simulink model "VisionProcessingDesign_UCS"  (R2025b)
settings: Solver=FixedStepDiscrete  StartTime=0.0  StopTime=tspan  FixedStep=dt_sim  RelTol=1e-3
undefined symbols (not defined in the file): camHardwareDistK, dt_sample, gate1_Pose, M_WorldToUCS, pathPoses, redSlalomPoses, rel_CamPose_B, rel_CamPose_B_UCS, rel_CamPose_L, rel_CamPose_L_UCS, rel_CamPose_R, rel_CamPose_R_UCS, searchRescueEmojiPose, Sim3dSensor, surveyRepairEmojiPose, whiteSlalomPoses
libraries: sim3dlib x30, visionsinks x12, sim3dcameralib x3
settings Model: Creator=Liam  LastModifiedBy=Liam
settings OptimizationCC: DefaultParameterBehavior=Inlined  EnhancedBackFolding=on  PassReuseOutputArgsThreshold=0.0  ZeroExternalMemoryAtStartup=off  ZeroInternalMemoryAtStartup=off  InitFltsAndDblsToZero=on  OptimizeBlockOrder=speed  DifferentSizesBufferReuse=on  OptimizationCustomize=off
settings DebuggingCC: ParameterTunabilityLossMsg=error
settings HardwareCC: ProdLongLongMode=on  TargetLongLongMode=on
settings SFSimCC: SimTargetLang=C++  SimDLTargetLibrary=mkl-dnn
settings RTWCC: GenCodeOnly=on  GenerateReport=on  Toolchain=NVIDIA CUDA (w/Microsoft Visual C++ 2022) | nmake (64-bit Windows)  LaunchReport=on  TargetLang=C++  GenerateGPUCode=CUDA
settings CodeAppCC: ForceParamTrailComments=on  OperatorAnnotations=on
settings GRTTargetCC: TargetLangStandard=C++11 (ISO)  MatFileLogging=off  CodeInterfacePackaging=C++ class  SubcomponentCodeInterfacePackaging=C++ class

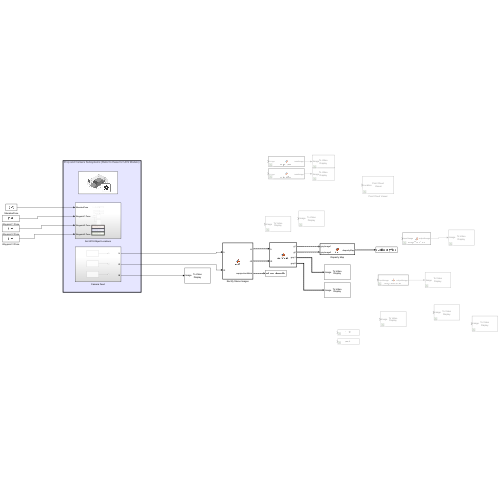
[thumbnail: Simulink's stored preview of the top-level diagram]
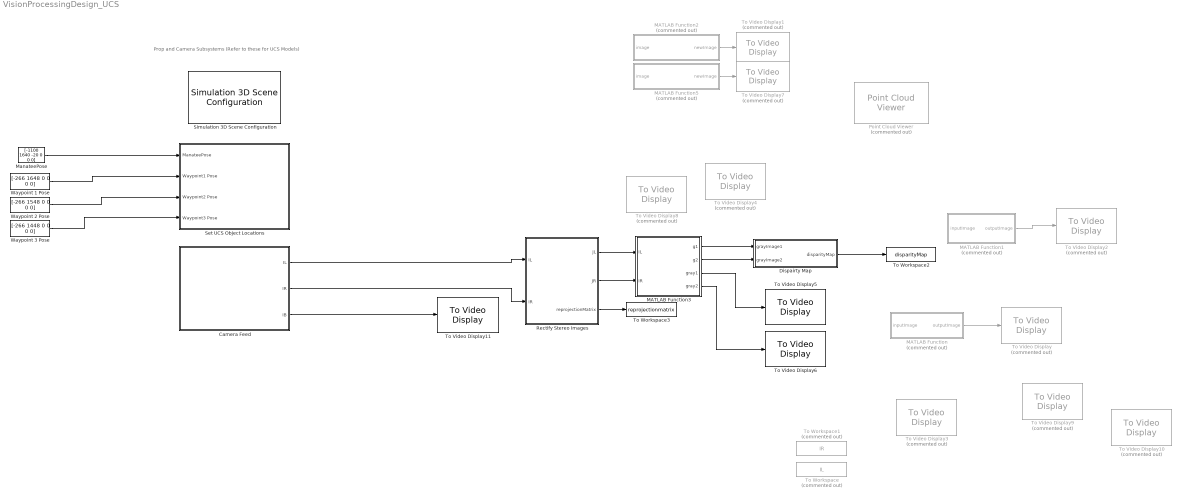
== system VisionProcessingDesign_UCS ==
  note: Prop and Camera Subsystems (Refer to these for UCS Models)
  Camera Feed : Subsystem  Priority=1
  Dispairty Map : MATLAB Function  TreatAsAtomicUnit=on
  MATLAB Function : MATLAB Function  Commented=on  TreatAsAtomicUnit=on
  MATLAB Function1 : MATLAB Function  Commented=on  TreatAsAtomicUnit=on
  MATLAB Function2 : MATLAB Function  Commented=on  TreatAsAtomicUnit=on
  MATLAB Function3 : MATLAB Function  TreatAsAtomicUnit=on
  MATLAB Function5 : MATLAB Function  Commented=on  TreatAsAtomicUnit=on
  ManateePose : Constant  Value=[-1100 1640 -20 0 0 0]
  Point Cloud Viewer : PointCloudViewer  Commented=on
  Rectify Stereo Images : MATLAB Function  TreatAsAtomicUnit=on
  Set UCS Object Locations : Subsystem  Priority=1
  Simulation 3D Scene Configuration : sim3dlib/Simulation 3D Scene Configuration  Priority=0  ProjectFormat=Unreal Executable  SceneDesc=Straight road  ProjectName=C:\Users\Liam\OneDrive\Documents\GitHub\SimulinkPlant\DROP UCS PACKAGED BUILD HERE\EllingtonPoolSim.exe  ScenePath=/Game/Olympic_Pool_Course  UEProjPath=C:\Users\Liam\OneDrive\Documents\GitHub\Vision_Sim\Unreal\UnrealProjects\SimulinkCoSimulation\EllingtonPoolSim\EllingtonPoolSim.uproject  EnableOpenDRIVE=off  vehTagList={'Custom';'Scene Origin'}  vehTag=Scene Origin  AttachedCameraRelativeTranslation=[0 0 0]  FreeCameraDefaultInitialTranslation=[-6, 0, 2]  AttachedCameraRelativeRotation=[0 0 0]  FreeCameraDefaultInitialRotation=[0, -15, 0]  ViewpointName=Custom  FreeCameraInitialTranslation=[0, 0, 0]  ViewpointTranslation=[0 0 0]  FreeCameraInitialRotation=[0, 0, 0]  ViewpointRotation=[0 0 0]  OpVisEn=off  Ts=dt_sample  EnableWindow=on  EnableRemoteAccess=off  EnableWeather=off  SunAzimuth=90  SunAltitude=40.0  EnableGeospatialSun=off  Latitude=0  Longitude=0  Date=2023-01-01  Time=10:30:00  GeoTimeZone=-5.0  SunDaylightSaving=off  wind=1  clouds=10  EnableVolumetricClouds=off  CloudCoverage=0  CloudAltitude=6  fog=0  rain=0  RaindropsEffect=off  SnowDensity=0  EnableGeospatial=off  TilesetSource=Earth terrain  UseTrueOrigin=off  OriginHeight=200  OriginLatitude=40.744652  OriginLongitude=-73.988864  MapStyle=Aerial  AdditionalAssetIDs=[]  UseAdvancedSunSky=off  SolarTime=11  TimeZone=-5  Day=21  Month=9  Year=2022  UseDaylightSavingTime=on  DSTStartDay=10  DSTStartMonth=3  DSTEndDay=3  DSTEndMonth=11  DSTSwitchHour=2  sensorTag=MainCamera1  sensorId=1  sensorName=MainCamera1  mountLoc=Origin  offsetFlag=off  tmountOffset=[0, 0, 0]  rmountOffset=[0, 0, 0]  HorizontalResolution=1280  VerticalResolution=720  HorizontalFOV=60  mountPoint=[0 0 0]  mountOrientation=[0 0 0]  aMode=3  ID=1  GeoTrigger=Inactive  ViewNameList={'Custom'}  ViewTranslationList={'[0 0 0]'}  ViewRotationList={'[0 0 0]'}
      settings: LibrarySourceBlock=drivingsim3d/Simulation 3D Scene Configuration
  To Video Display{,1..3,7,9..10} (7 alike) : visionsinks/To Video Display  Commented=on  windowSizeMode=Normal  openAtMdlStart=on  fullScreen=off  videoWindowX=536805376  videoWindowY=536805376  saveWindowSize=off  videoWindowWidth=1920  videoWindowHeight=1080  inputColorFormat=RGB  inputType=Obsolete  imagePorts=One multidimensional signal  OutputDevice=On-screen video monitor  dataOrg=Column-major  isWindowOpen=off
  To Video Display11 : visionsinks/To Video Display  windowSizeMode=Normal  openAtMdlStart=on  fullScreen=off  videoWindowX=536805376  videoWindowY=536805376  saveWindowSize=off  videoWindowWidth=1920  videoWindowHeight=1080  inputColorFormat=RGB  inputType=Obsolete  imagePorts=One multidimensional signal  OutputDevice=On-screen video monitor  dataOrg=Column-major  isWindowOpen=off
  To Video Display4 : visionsinks/To Video Display  Commented=on  windowSizeMode=Normal  openAtMdlStart=on  fullScreen=off  videoWindowX=536805376  videoWindowY=536805376  saveWindowSize=off  videoWindowWidth=1491  videoWindowHeight=834  inputColorFormat=RGB  inputType=Obsolete  imagePorts=One multidimensional signal  OutputDevice=On-screen video monitor  dataOrg=Column-major  isWindowOpen=off
  To Video Display5 : visionsinks/To Video Display  windowSizeMode=Normal  openAtMdlStart=on  fullScreen=off  videoWindowX=536805376  videoWindowY=536805376  saveWindowSize=off  videoWindowWidth=1491  videoWindowHeight=834  inputColorFormat=RGB  inputType=Obsolete  imagePorts=One multidimensional signal  OutputDevice=On-screen video monitor  dataOrg=Column-major  isWindowOpen=off
  To Video Display6 : visionsinks/To Video Display  windowSizeMode=Normal  openAtMdlStart=on  fullScreen=off  videoWindowX=536805376  videoWindowY=536805376  saveWindowSize=off  videoWindowWidth=1491  videoWindowHeight=834  inputColorFormat=RGB  inputType=Obsolete  imagePorts=One multidimensional signal  OutputDevice=On-screen video monitor  dataOrg=Column-major  isWindowOpen=off
  To Video Display8 : visionsinks/To Video Display  Commented=on  windowSizeMode=Normal  openAtMdlStart=on  fullScreen=off  videoWindowX=536805376  videoWindowY=536805376  saveWindowSize=off  videoWindowWidth=1491  videoWindowHeight=834  inputColorFormat=RGB  inputType=Obsolete  imagePorts=One multidimensional signal  OutputDevice=On-screen video monitor  dataOrg=Column-major  isWindowOpen=off
  To Workspace : ToWorkspace  Commented=on  VariableName=IL  SaveFormat=Structure  SampleTime=-1
  To Workspace1 : ToWorkspace  Commented=on  VariableName=IR  SaveFormat=Structure  SampleTime=-1
  To Workspace2 : ToWorkspace  VariableName=disparityMap  SaveFormat=Structure  SampleTime=-1
  To Workspace3 : ToWorkspace  VariableName=reprojectionmatrix  SaveFormat=Structure  SampleTime=-1
  Waypoint 1 Pose : Constant  Value=[-266 1648 0 0 0 0]
  Waypoint 2 Pose : Constant  Value=[-266 1548 0 0 0 0]
  Waypoint 3 Pose : Constant  Value=[-266 1448 0 0 0 0]
  wires:
  ManateePose/1 -> Set UCS Object Locations/1(ManateePose)
  MATLAB Function/1(outputImage) -> To Video Display/1
  MATLAB Function1/1(outputImage) -> To Video Display2/1
  MATLAB Function2/1(newImage) -> To Video Display1/1
  MATLAB Function5/1(newImage) -> To Video Display7/1
  Camera Feed/1(IL) -> Rectify Stereo Images/1(IL)
  Camera Feed/2(IR) -> Rectify Stereo Images/2(IR)
  Camera Feed/3(IB) -> To Video Display11/1
  Waypoint 1 Pose/1 -> Set UCS Object Locations/2(Waypoint1 Pose)
  Waypoint 2 Pose/1 -> Set UCS Object Locations/3(Waypoint2 Pose)
  Waypoint 3 Pose/1 -> Set UCS Object Locations/4(Waypoint3 Pose)
  MATLAB Function3/2(g2) -> Dispairty Map/2(grayImage2)
  Rectify Stereo Images/1(JL) -> MATLAB Function3/1(IL)
  MATLAB Function3/1(g1) -> Dispairty Map/1(grayImage1)
  Rectify Stereo Images/2(JR) -> MATLAB Function3/2(IR)
  Dispairty Map/1(disparityMap) -> To Workspace2/1
  MATLAB Function3/3(gray1) -> To Video Display5/1
  MATLAB Function3/4(gray2) -> To Video Display6/1
  Rectify Stereo Images/3(reprojectionMatrix) -> To Workspace3/1

== system VisionProcessingDesign_UCS/Camera Feed ==
  Simulation 3D Manatee Bottom Camera : sim3dcameralib/Simulation 3D Camera  Priority=1  sensorTag=Sim3dSensor�  sensorId=1  sensorName=Sim3dSensor�  vehTagList={'Scene Origin'}  vehTag=Scene Origin  CoordinateSystem=Default  mountLoc=Origin  offsetFlag=on  tmountOffset=rel_CamPose_B_UCS(1:3) / 100  extTmount=off  rmountOffset=rel_CamPose_B(4:6)  extRmount=off  FocalLength=[2.97 / 0.0028, 2.97 / 0.0028]  OpticalCenter=[960, 540]  ImageSize=[1080, 1920]  RadialDistortion=[camHardwareDistK(1) camHardwareDistK(2) camHardwareDistK(5)]  TangentialDistortion=[camHardwareDistK(3) camHardwareDistK(4)]  SensorSkew=0  VisualizeFieldOfView=on  FieldOfViewRange=61  DepthOutportEnabled=off  SemanticOutportEnabled=off  TransformOutportEnabled=off  SampleTime=dt_sample  mountPoint=[0.23 0 -0.08]  mountOrientation=[0 -1.5707963267949 0]  aMode=5  ID=1
      settings: LibrarySourceBlock=sl3dlib/Simulation 3D/Sensors/Simulation 3D Camera
  Simulation 3D Manatee Left Camera : sim3dcameralib/Simulation 3D Camera  Priority=1  sensorTag=Sim3dSensor�  sensorId=2  sensorName=Sim3dSensor�  vehTagList={'Scene Origin'}  vehTag=Scene Origin  CoordinateSystem=Default  mountLoc=Origin  offsetFlag=on  tmountOffset=rel_CamPose_L_UCS(1:3) / 100  extTmount=off  rmountOffset=rel_CamPose_L(4:6)  extRmount=off  FocalLength=[2.97 / 0.0028, 2.97 / 0.0028]  OpticalCenter=[960, 540]  ImageSize=[1080, 1920]  RadialDistortion=[camHardwareDistK(1) camHardwareDistK(2) camHardwareDistK(5)]  TangentialDistortion=[camHardwareDistK(3) camHardwareDistK(4)]  SensorSkew=0  VisualizeFieldOfView=on  FieldOfViewRange=61  DepthOutportEnabled=off  SemanticOutportEnabled=off  TransformOutportEnabled=off  SampleTime=dt_sample  mountPoint=[0.38 -0.024 0.14]  mountOrientation=[0 0 0]  aMode=5  ID=2
      settings: LibrarySourceBlock=sl3dlib/Simulation 3D/Sensors/Simulation 3D Camera
  Simulation 3D Manatee Right Camera : sim3dcameralib/Simulation 3D Camera  Priority=1  sensorTag=Sim3dSensor�  sensorId=3  sensorName=Sim3dSensor�  vehTagList={'Scene Origin'}  vehTag=Scene Origin  CoordinateSystem=Default  mountLoc=Origin  offsetFlag=on  tmountOffset=rel_CamPose_R_UCS(1:3) / 100  extTmount=off  rmountOffset=rel_CamPose_R(4:6)  extRmount=off  FocalLength=[2.97 / 0.0028, 2.97 / 0.0028]  OpticalCenter=[960, 540]  ImageSize=[1080, 1920]  RadialDistortion=[camHardwareDistK(1) camHardwareDistK(2) camHardwareDistK(5)]  TangentialDistortion=[camHardwareDistK(3) camHardwareDistK(4)]  SensorSkew=0  VisualizeFieldOfView=on  FieldOfViewRange=61  DepthOutportEnabled=off  SemanticOutportEnabled=off  TransformOutportEnabled=off  SampleTime=dt_sample  mountPoint=[0.38 0.024 0.14]  mountOrientation=[0 0 0]  aMode=5  ID=3
      settings: LibrarySourceBlock=sl3dlib/Simulation 3D/Sensors/Simulation 3D Camera
  IL : Outport
  IR : Outport  Port=2
  IB : Outport  Port=3
  wires:
  Simulation 3D Manatee Left Camera/1 -> IL/1
  Simulation 3D Manatee Right Camera/1 -> IR/1
  Simulation 3D Manatee Bottom Camera/1 -> IB/1

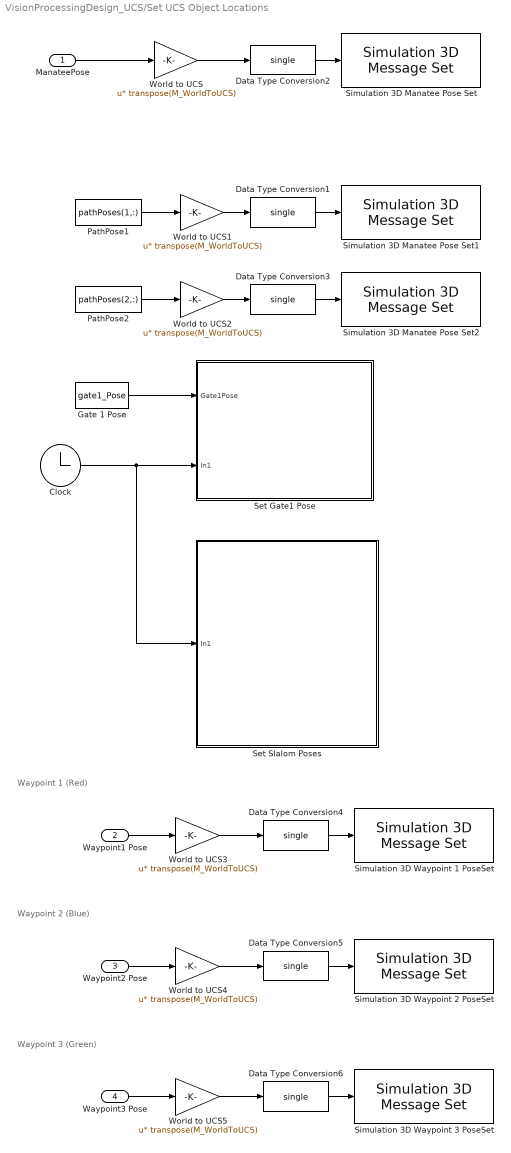
== system VisionProcessingDesign_UCS/Set UCS Object Locations ==
  note: Waypoint 1 (Red)
  note: Waypoint 2 (Blue)
  note: Waypoint 3 (Green)
  ManateePose : Inport
  Waypoint1 Pose : Inport  Port=2
  Waypoint2 Pose : Inport  Port=3
  Waypoint3 Pose : Inport  Port=4
  Clock : Clock
      settings: Decimation=dt_sample/dt_sim
  Data Type Conversion{1..6} (6 alike) : DataTypeConversion  OutDataTypeStr=single  SaturateOnIntegerOverflow=off  RndMeth=Floor
  Gate 1 Pose : Constant  Value=gate1_Pose
  PathPose1 : Constant  Value=pathPoses(1,:)
  PathPose2 : Constant  Value=pathPoses(2,:)
  Set Gate1 Pose : Subsystem
  Set Slalom Poses : Subsystem
  Simulation 3D Manatee Pose Set : sim3dlib/Simulation 3D Message Set  Priority=-1  SigName=ManateePoseSet  Ts=dt_sample  aMode=0
      settings: LibrarySourceBlock=aerolibsim3d/Simulation 3D Message Set
  Simulation 3D Manatee Pose Set1 : sim3dlib/Simulation 3D Message Set  Priority=-1  SigName=Path1PoseSet  Ts=dt_sample  aMode=0
      settings: LibrarySourceBlock=aerolibsim3d/Simulation 3D Message Set
  Simulation 3D Manatee Pose Set2 : sim3dlib/Simulation 3D Message Set  Priority=-1  SigName=Path2PoseSet  Ts=dt_sample  aMode=0
      settings: LibrarySourceBlock=aerolibsim3d/Simulation 3D Message Set
  Simulation 3D Waypoint 1 PoseSet : sim3dlib/Simulation 3D Message Set  Priority=-1  SigName=Waypoint1PoseSet  Ts=dt_sample  aMode=0
      settings: LibrarySourceBlock=aerolibsim3d/Simulation 3D Message Set
  Simulation 3D Waypoint 2 PoseSet : sim3dlib/Simulation 3D Message Set  Priority=-1  SigName=Waypoint2PoseSet  Ts=dt_sample  aMode=0
      settings: LibrarySourceBlock=aerolibsim3d/Simulation 3D Message Set
  Simulation 3D Waypoint 3 PoseSet : sim3dlib/Simulation 3D Message Set  Priority=-1  SigName=Waypoint3PoseSet  Ts=dt_sample  aMode=0
      settings: LibrarySourceBlock=aerolibsim3d/Simulation 3D Message Set
  World to UCS{,1..5} (6 alike) : Gain  Gain=transpose(M_WorldToUCS)  Multiplication=Matrix(u*K)
  wires:
  Gate 1 Pose/1 -> Set Gate1 Pose/1(Gate1Pose)
  Data Type Conversion2/1 -> Simulation 3D Manatee Pose Set/1
  World to UCS1/1 -> Data Type Conversion1/1
  Data Type Conversion1/1 -> Simulation 3D Manatee Pose Set1/1
  PathPose1/1 -> World to UCS1/1
  World to UCS2/1 -> Data Type Conversion3/1
  Data Type Conversion3/1 -> Simulation 3D Manatee Pose Set2/1
  PathPose2/1 -> World to UCS2/1
  Clock/1 -> Set Slalom Poses/1(In1), Set Gate1 Pose/2(In1)
  World to UCS/1 -> Data Type Conversion2/1
  ManateePose/1 -> World to UCS/1
  Waypoint1 Pose/1 -> World to UCS3/1
  Data Type Conversion4/1 -> Simulation 3D Waypoint 1 PoseSet/1
  World to UCS3/1 -> Data Type Conversion4/1
  Waypoint2 Pose/1 -> World to UCS4/1
  Data Type Conversion5/1 -> Simulation 3D Waypoint 2 PoseSet/1
  World to UCS4/1 -> Data Type Conversion5/1
  World to UCS5/1 -> Data Type Conversion6/1
  Waypoint3 Pose/1 -> World to UCS5/1
  Data Type Conversion6/1 -> Simulation 3D Waypoint 3 PoseSet/1

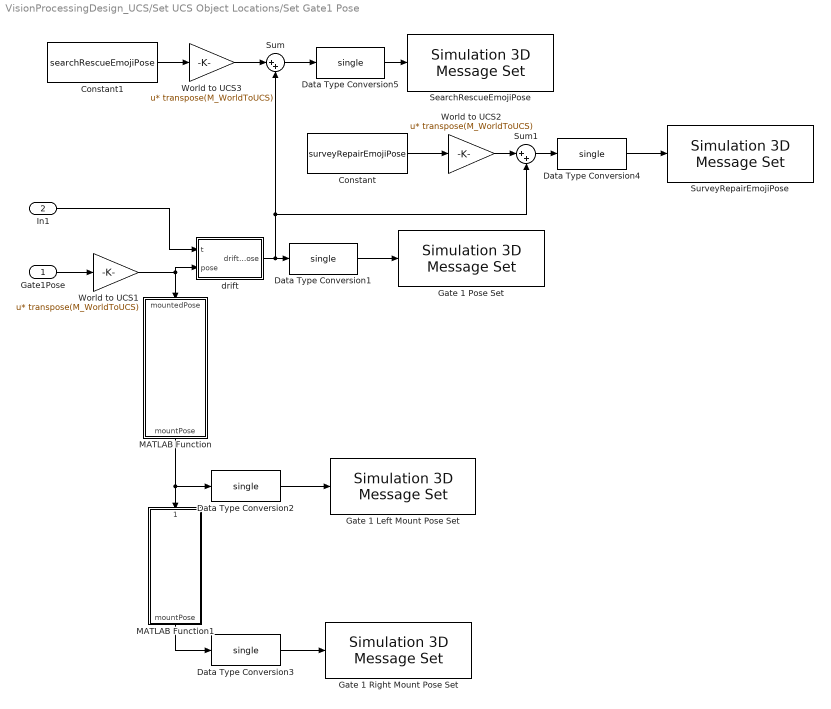
== system VisionProcessingDesign_UCS/Set UCS Object Locations/Set Gate1 Pose ==
  Gate1Pose : Inport
  In1 : Inport  Port=2
  Constant : Constant  Value=surveyRepairEmojiPose
  Constant1 : Constant  Value=searchRescueEmojiPose
  Data Type Conversion{1..5} (5 alike) : DataTypeConversion  OutDataTypeStr=single  SaturateOnIntegerOverflow=off  RndMeth=Floor
  Gate 1 Left Mount Pose Set : sim3dlib/Simulation 3D Message Set  Priority=-1  SigName=Gate1LeftMountPoseSet  Ts=dt_sample  aMode=0
      settings: LibrarySourceBlock=aerolibsim3d/Simulation 3D Message Set
  Gate 1 Pose Set : sim3dlib/Simulation 3D Message Set  Priority=-1  SigName=Gate1PoseSet  Ts=dt_sample  aMode=0
      settings: LibrarySourceBlock=aerolibsim3d/Simulation 3D Message Set
  Gate 1 Right Mount Pose Set : sim3dlib/Simulation 3D Message Set  Priority=-1  SigName=Gate1RightMountPoseSet  Ts=dt_sample  aMode=0
      settings: LibrarySourceBlock=aerolibsim3d/Simulation 3D Message Set
  MATLAB Function : MATLAB Function  TreatAsAtomicUnit=on
  MATLAB Function1 : MATLAB Function  TreatAsAtomicUnit=on
  SearchRescueEmojiPose : sim3dlib/Simulation 3D Message Set  Priority=-1  SigName=SearchRescueEmojiPoseSet  Ts=dt_sample  aMode=0
      settings: LibrarySourceBlock=aerolibsim3d/Simulation 3D Message Set
  Sum : Sum  Inputs=|++
  Sum1 : Sum  Inputs=|++
  SurveyRepairEmojiPose : sim3dlib/Simulation 3D Message Set  Priority=-1  SigName=SurveyRepairEmojiPoseSet  Ts=dt_sample  aMode=0
      settings: LibrarySourceBlock=aerolibsim3d/Simulation 3D Message Set
  World to UCS1 : Gain  Gain=transpose(M_WorldToUCS)  Multiplication=Matrix(u*K)
  World to UCS2 : Gain  Gain=transpose(M_WorldToUCS)  Multiplication=Matrix(u*K)
  World to UCS3 : Gain  Gain=transpose(M_WorldToUCS)  Multiplication=Matrix(u*K)
  drift : MATLAB Function  TreatAsAtomicUnit=on
  wires:
  Gate1Pose/1 -> World to UCS1/1
  MATLAB Function/1(mountPose) -> Data Type Conversion2/1, MATLAB Function1/1(leftMountPose)
  Data Type Conversion2/1 -> Gate 1 Left Mount Pose Set/1
  Data Type Conversion3/1 -> Gate 1 Right Mount Pose Set/1
  Data Type Conversion1/1 -> Gate 1 Pose Set/1
  World to UCS1/1 -> drift/2(pose), MATLAB Function/1(mountedPose)
  MATLAB Function1/1(mountPose) -> Data Type Conversion3/1
  Data Type Conversion4/1 -> SurveyRepairEmojiPose/1
  Constant/1 -> World to UCS2/1
  Data Type Conversion5/1 -> SearchRescueEmojiPose/1
  Constant1/1 -> World to UCS3/1
  Sum/1 -> Data Type Conversion5/1
  World to UCS3/1 -> Sum/1
  World to UCS2/1 -> Sum1/1
  Sum1/1 -> Data Type Conversion4/1
  In1/1 -> drift/1(t)
  drift/1(driftPose) -> Data Type Conversion1/1, Sum1/2, Sum/2

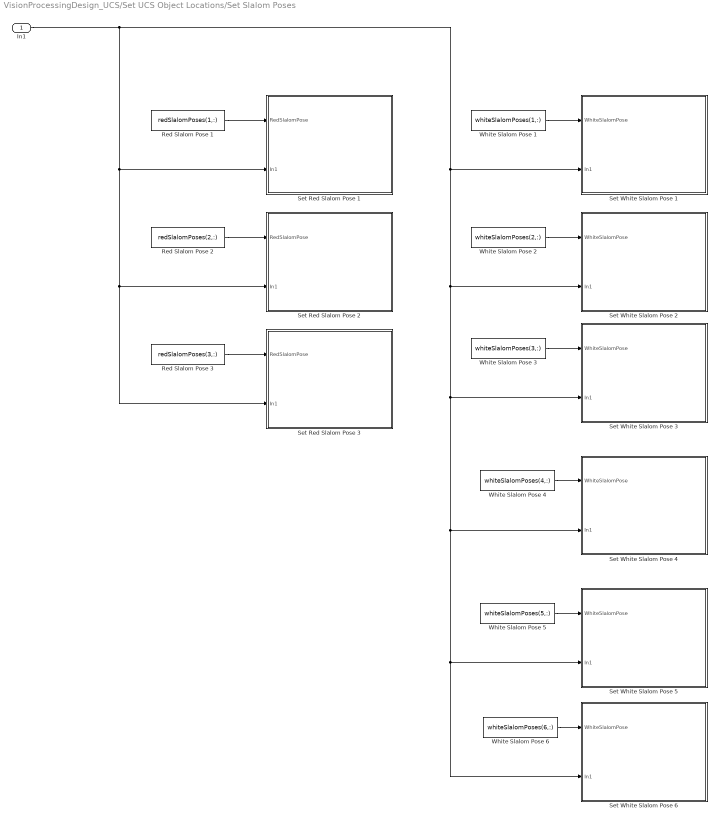
== system VisionProcessingDesign_UCS/Set UCS Object Locations/Set Slalom Poses ==
  In1 : Inport
  Red Slalom Pose 1 : Constant  Value=redSlalomPoses(1,:)
  Red Slalom Pose 2 : Constant  Value=redSlalomPoses(2,:)
  Red Slalom Pose 3 : Constant  Value=redSlalomPoses(3,:)
  Set Red Slalom Pose 1 : Subsystem
  Set Red Slalom Pose 2 : Subsystem
  Set Red Slalom Pose 3 : Subsystem
  Set White Slalom Pose 1 : Subsystem
  Set White Slalom Pose 2 : Subsystem
  Set White Slalom Pose 3 : Subsystem
  Set White Slalom Pose 4 : Subsystem
  Set White Slalom Pose 5 : Subsystem
  Set White Slalom Pose 6 : Subsystem
  White Slalom Pose 1 : Constant  Value=whiteSlalomPoses(1,:)
  White Slalom Pose 2 : Constant  Value=whiteSlalomPoses(2,:)
  White Slalom Pose 3 : Constant  Value=whiteSlalomPoses(3,:)
  White Slalom Pose 4 : Constant  Value=whiteSlalomPoses(4,:)
  White Slalom Pose 5 : Constant  Value=whiteSlalomPoses(5,:)
  White Slalom Pose 6 : Constant  Value=whiteSlalomPoses(6,:)
  wires:
  Red Slalom Pose 1/1 -> Set Red Slalom Pose 1/1(RedSlalomPose)
  Red Slalom Pose 2/1 -> Set Red Slalom Pose 2/1(RedSlalomPose)
  Red Slalom Pose 3/1 -> Set Red Slalom Pose 3/1(RedSlalomPose)
  White Slalom Pose 1/1 -> Set White Slalom Pose 1/1(WhiteSlalomPose)
  White Slalom Pose 2/1 -> Set White Slalom Pose 2/1(WhiteSlalomPose)
  White Slalom Pose 3/1 -> Set White Slalom Pose 3/1(WhiteSlalomPose)
  White Slalom Pose 4/1 -> Set White Slalom Pose 4/1(WhiteSlalomPose)
  White Slalom Pose 5/1 -> Set White Slalom Pose 5/1(WhiteSlalomPose)
  White Slalom Pose 6/1 -> Set White Slalom Pose 6/1(WhiteSlalomPose)
  In1/1 -> Set Red Slalom Pose 3/2(In1), Set Red Slalom Pose 2/2(In1), Set Red Slalom Pose 1/2(In1), Set White Slalom Pose 6/2(In1), Set White Slalom Pose 5/2(In1), Set White Slalom Pose 4/2(In1), Set White Slalom Pose 3/2(In1), Set White Slalom Pose 2/2(In1), Set White Slalom Pose 1/2(In1)

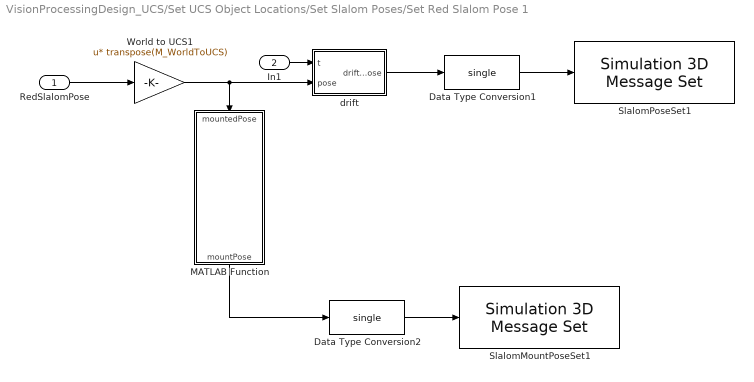
== system VisionProcessingDesign_UCS/Set UCS Object Locations/Set Slalom Poses/Set Red Slalom Pose 1 ==
  RedSlalomPose : Inport
  In1 : Inport  Port=2
  Data Type Conversion1 : DataTypeConversion  OutDataTypeStr=single  SaturateOnIntegerOverflow=off  RndMeth=Floor
  Data Type Conversion2 : DataTypeConversion  OutDataTypeStr=single  SaturateOnIntegerOverflow=off  RndMeth=Floor
  MATLAB Function : MATLAB Function  TreatAsAtomicUnit=on
  SlalomMountPoseSet1 : sim3dlib/Simulation 3D Message Set  Priority=-1  SigName=RedSlalom1MountPoseSet  Ts=dt_sample  aMode=0
      settings: LibrarySourceBlock=aerolibsim3d/Simulation 3D Message Set
  SlalomPoseSet1 : sim3dlib/Simulation 3D Message Set  Priority=-1  SigName=RedSlalom1PoseSet  Ts=dt_sample  aMode=0
      settings: LibrarySourceBlock=aerolibsim3d/Simulation 3D Message Set
  World to UCS1 : Gain  Gain=transpose(M_WorldToUCS)  Multiplication=Matrix(u*K)
  drift : MATLAB Function  TreatAsAtomicUnit=on
  wires:
  RedSlalomPose/1 -> World to UCS1/1
  MATLAB Function/1(mountPose) -> Data Type Conversion2/1
  Data Type Conversion2/1 -> SlalomMountPoseSet1/1
  Data Type Conversion1/1 -> SlalomPoseSet1/1
  World to UCS1/1 -> drift/2(pose), MATLAB Function/1(mountedPose)
  drift/1(driftPose) -> Data Type Conversion1/1
  In1/1 -> drift/1(t)

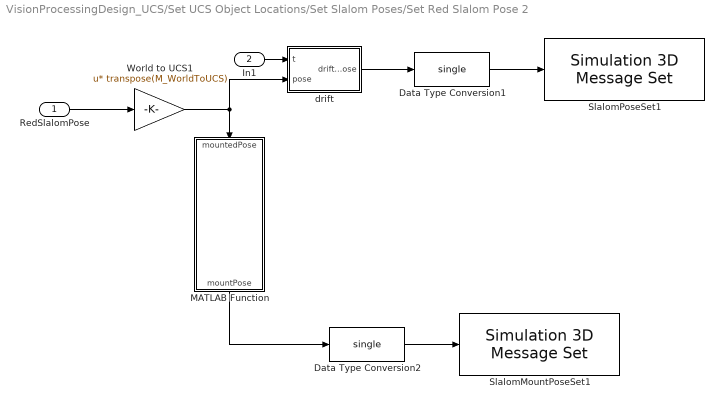
== system VisionProcessingDesign_UCS/Set UCS Object Locations/Set Slalom Poses/Set Red Slalom Pose 2 ==
  RedSlalomPose : Inport
  In1 : Inport  Port=2
  Data Type Conversion1 : DataTypeConversion  OutDataTypeStr=single  SaturateOnIntegerOverflow=off  RndMeth=Floor
  Data Type Conversion2 : DataTypeConversion  OutDataTypeStr=single  SaturateOnIntegerOverflow=off  RndMeth=Floor
  MATLAB Function : MATLAB Function  TreatAsAtomicUnit=on
  SlalomMountPoseSet1 : sim3dlib/Simulation 3D Message Set  Priority=-1  SigName=RedSlalom2MountPoseSet  Ts=dt_sample  aMode=0
      settings: LibrarySourceBlock=aerolibsim3d/Simulation 3D Message Set
  SlalomPoseSet1 : sim3dlib/Simulation 3D Message Set  Priority=-1  SigName=RedSlalom2PoseSet  Ts=dt_sample  aMode=0
      settings: LibrarySourceBlock=aerolibsim3d/Simulation 3D Message Set
  World to UCS1 : Gain  Gain=transpose(M_WorldToUCS)  Multiplication=Matrix(u*K)
  drift : MATLAB Function  TreatAsAtomicUnit=on
  wires:
  RedSlalomPose/1 -> World to UCS1/1
  MATLAB Function/1(mountPose) -> Data Type Conversion2/1
  Data Type Conversion2/1 -> SlalomMountPoseSet1/1
  Data Type Conversion1/1 -> SlalomPoseSet1/1
  World to UCS1/1 -> MATLAB Function/1(mountedPose), drift/2(pose)
  In1/1 -> drift/1(t)
  drift/1(driftPose) -> Data Type Conversion1/1

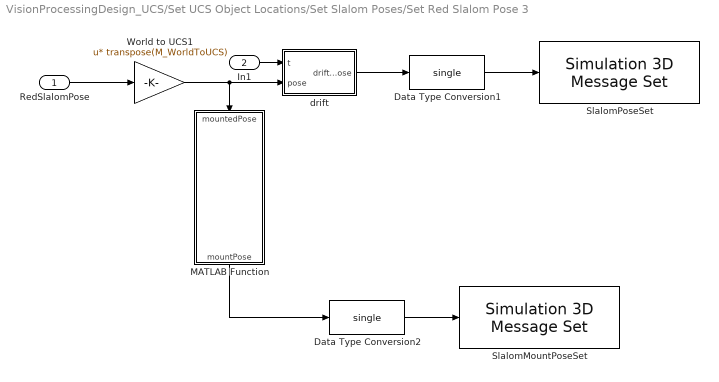
== system VisionProcessingDesign_UCS/Set UCS Object Locations/Set Slalom Poses/Set Red Slalom Pose 3 ==
  RedSlalomPose : Inport
  In1 : Inport  Port=2
  Data Type Conversion1 : DataTypeConversion  OutDataTypeStr=single  SaturateOnIntegerOverflow=off  RndMeth=Floor
  Data Type Conversion2 : DataTypeConversion  OutDataTypeStr=single  SaturateOnIntegerOverflow=off  RndMeth=Floor
  MATLAB Function : MATLAB Function  TreatAsAtomicUnit=on
  SlalomMountPoseSet : sim3dlib/Simulation 3D Message Set  Priority=-1  SigName=RedSlalom3MountPoseSet  Ts=dt_sample  aMode=0
      settings: LibrarySourceBlock=aerolibsim3d/Simulation 3D Message Set
  SlalomPoseSet : sim3dlib/Simulation 3D Message Set  Priority=-1  SigName=RedSlalom3PoseSet  Ts=dt_sample  aMode=0
      settings: LibrarySourceBlock=aerolibsim3d/Simulation 3D Message Set
  World to UCS1 : Gain  Gain=transpose(M_WorldToUCS)  Multiplication=Matrix(u*K)
  drift : MATLAB Function  TreatAsAtomicUnit=on
  wires:
  RedSlalomPose/1 -> World to UCS1/1
  MATLAB Function/1(mountPose) -> Data Type Conversion2/1
  Data Type Conversion2/1 -> SlalomMountPoseSet/1
  Data Type Conversion1/1 -> SlalomPoseSet/1
  World to UCS1/1 -> drift/2(pose), MATLAB Function/1(mountedPose)
  In1/1 -> drift/1(t)
  drift/1(driftPose) -> Data Type Conversion1/1

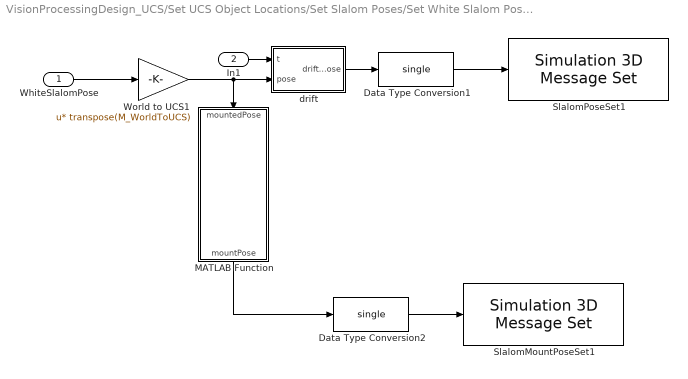
== system VisionProcessingDesign_UCS/Set UCS Object Locations/Set Slalom Poses/Set White Slalom Pose 1 ==
  WhiteSlalomPose : Inport
  In1 : Inport  Port=2
  Data Type Conversion1 : DataTypeConversion  OutDataTypeStr=single  SaturateOnIntegerOverflow=off  RndMeth=Floor
  Data Type Conversion2 : DataTypeConversion  OutDataTypeStr=single  SaturateOnIntegerOverflow=off  RndMeth=Floor
  MATLAB Function : MATLAB Function  TreatAsAtomicUnit=on
  SlalomMountPoseSet1 : sim3dlib/Simulation 3D Message Set  Priority=-1  SigName=WhiteSlalom1MountPoseSet  Ts=dt_sample  aMode=0
      settings: LibrarySourceBlock=aerolibsim3d/Simulation 3D Message Set
  SlalomPoseSet1 : sim3dlib/Simulation 3D Message Set  Priority=-1  SigName=WhiteSlalom1PoseSet  Ts=dt_sample  aMode=0
      settings: LibrarySourceBlock=aerolibsim3d/Simulation 3D Message Set
  World to UCS1 : Gain  Gain=transpose(M_WorldToUCS)  Multiplication=Matrix(u*K)
  drift : MATLAB Function  TreatAsAtomicUnit=on
  wires:
  WhiteSlalomPose/1 -> World to UCS1/1
  MATLAB Function/1(mountPose) -> Data Type Conversion2/1
  Data Type Conversion2/1 -> SlalomMountPoseSet1/1
  Data Type Conversion1/1 -> SlalomPoseSet1/1
  World to UCS1/1 -> drift/2(pose), MATLAB Function/1(mountedPose)
  In1/1 -> drift/1(t)
  drift/1(driftPose) -> Data Type Conversion1/1

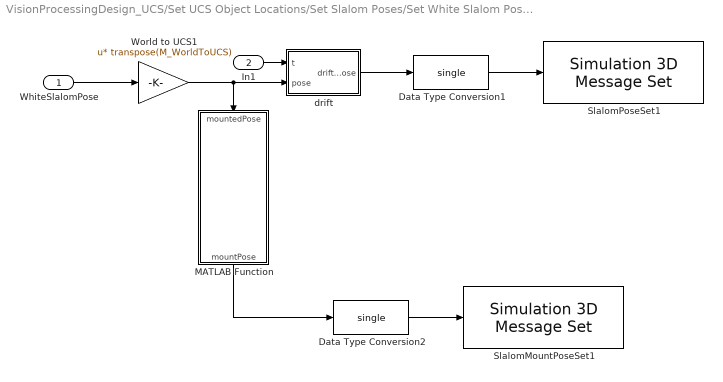
== system VisionProcessingDesign_UCS/Set UCS Object Locations/Set Slalom Poses/Set White Slalom Pose 2 ==
  WhiteSlalomPose : Inport
  In1 : Inport  Port=2
  Data Type Conversion1 : DataTypeConversion  OutDataTypeStr=single  SaturateOnIntegerOverflow=off  RndMeth=Floor
  Data Type Conversion2 : DataTypeConversion  OutDataTypeStr=single  SaturateOnIntegerOverflow=off  RndMeth=Floor
  MATLAB Function : MATLAB Function  TreatAsAtomicUnit=on
  SlalomMountPoseSet1 : sim3dlib/Simulation 3D Message Set  Priority=-1  SigName=WhiteSlalom2MountPoseSet  Ts=dt_sample  aMode=0
      settings: LibrarySourceBlock=aerolibsim3d/Simulation 3D Message Set
  SlalomPoseSet1 : sim3dlib/Simulation 3D Message Set  Priority=-1  SigName=WhiteSlalom2PoseSet  Ts=dt_sample  aMode=0
      settings: LibrarySourceBlock=aerolibsim3d/Simulation 3D Message Set
  World to UCS1 : Gain  Gain=transpose(M_WorldToUCS)  Multiplication=Matrix(u*K)
  drift : MATLAB Function  TreatAsAtomicUnit=on
  wires:
  WhiteSlalomPose/1 -> World to UCS1/1
  MATLAB Function/1(mountPose) -> Data Type Conversion2/1
  Data Type Conversion2/1 -> SlalomMountPoseSet1/1
  Data Type Conversion1/1 -> SlalomPoseSet1/1
  World to UCS1/1 -> drift/2(pose), MATLAB Function/1(mountedPose)
  In1/1 -> drift/1(t)
  drift/1(driftPose) -> Data Type Conversion1/1

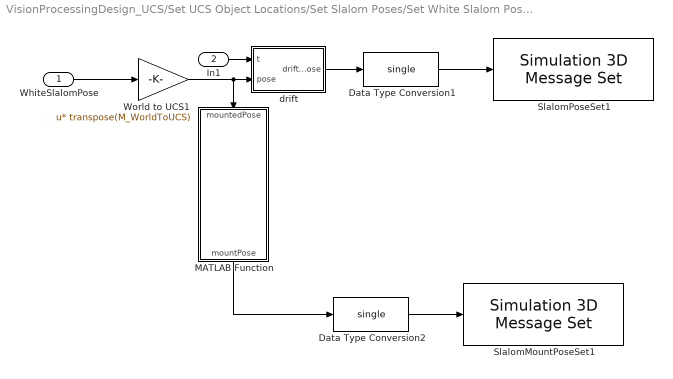
== system VisionProcessingDesign_UCS/Set UCS Object Locations/Set Slalom Poses/Set White Slalom Pose 3 ==
  WhiteSlalomPose : Inport
  In1 : Inport  Port=2
  Data Type Conversion1 : DataTypeConversion  OutDataTypeStr=single  SaturateOnIntegerOverflow=off  RndMeth=Floor
  Data Type Conversion2 : DataTypeConversion  OutDataTypeStr=single  SaturateOnIntegerOverflow=off  RndMeth=Floor
  MATLAB Function : MATLAB Function  TreatAsAtomicUnit=on
  SlalomMountPoseSet1 : sim3dlib/Simulation 3D Message Set  Priority=-1  SigName=WhiteSlalom3MountPoseSet  Ts=dt_sample  aMode=0
      settings: LibrarySourceBlock=aerolibsim3d/Simulation 3D Message Set
  SlalomPoseSet1 : sim3dlib/Simulation 3D Message Set  Priority=-1  SigName=WhiteSlalom3PoseSet  Ts=dt_sample  aMode=0
      settings: LibrarySourceBlock=aerolibsim3d/Simulation 3D Message Set
  World to UCS1 : Gain  Gain=transpose(M_WorldToUCS)  Multiplication=Matrix(u*K)
  drift : MATLAB Function  TreatAsAtomicUnit=on
  wires:
  WhiteSlalomPose/1 -> World to UCS1/1
  MATLAB Function/1(mountPose) -> Data Type Conversion2/1
  Data Type Conversion2/1 -> SlalomMountPoseSet1/1
  Data Type Conversion1/1 -> SlalomPoseSet1/1
  World to UCS1/1 -> drift/2(pose), MATLAB Function/1(mountedPose)
  In1/1 -> drift/1(t)
  drift/1(driftPose) -> Data Type Conversion1/1

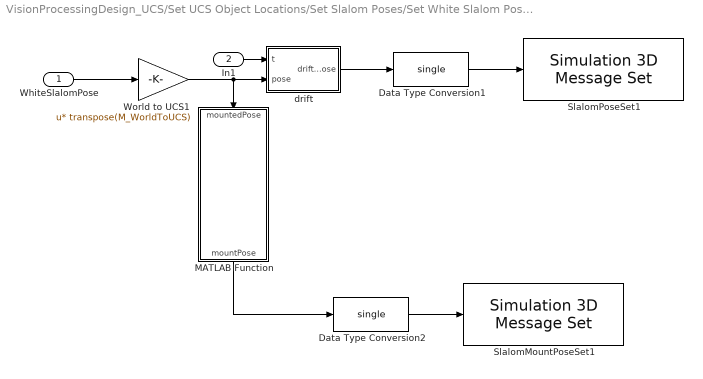
== system VisionProcessingDesign_UCS/Set UCS Object Locations/Set Slalom Poses/Set White Slalom Pose 4 ==
  WhiteSlalomPose : Inport
  In1 : Inport  Port=2
  Data Type Conversion1 : DataTypeConversion  OutDataTypeStr=single  SaturateOnIntegerOverflow=off  RndMeth=Floor
  Data Type Conversion2 : DataTypeConversion  OutDataTypeStr=single  SaturateOnIntegerOverflow=off  RndMeth=Floor
  MATLAB Function : MATLAB Function  TreatAsAtomicUnit=on
  SlalomMountPoseSet1 : sim3dlib/Simulation 3D Message Set  Priority=-1  SigName=WhiteSlalom4MountPoseSet  Ts=dt_sample  aMode=0
      settings: LibrarySourceBlock=aerolibsim3d/Simulation 3D Message Set
  SlalomPoseSet1 : sim3dlib/Simulation 3D Message Set  Priority=-1  SigName=WhiteSlalom4PoseSet  Ts=dt_sample  aMode=0
      settings: LibrarySourceBlock=aerolibsim3d/Simulation 3D Message Set
  World to UCS1 : Gain  Gain=transpose(M_WorldToUCS)  Multiplication=Matrix(u*K)
  drift : MATLAB Function  TreatAsAtomicUnit=on
  wires:
  WhiteSlalomPose/1 -> World to UCS1/1
  MATLAB Function/1(mountPose) -> Data Type Conversion2/1
  Data Type Conversion2/1 -> SlalomMountPoseSet1/1
  Data Type Conversion1/1 -> SlalomPoseSet1/1
  World to UCS1/1 -> drift/2(pose), MATLAB Function/1(mountedPose)
  In1/1 -> drift/1(t)
  drift/1(driftPose) -> Data Type Conversion1/1

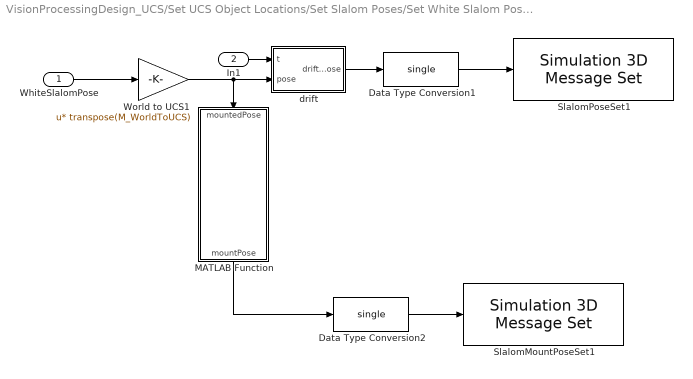
== system VisionProcessingDesign_UCS/Set UCS Object Locations/Set Slalom Poses/Set White Slalom Pose 5 ==
  WhiteSlalomPose : Inport
  In1 : Inport  Port=2
  Data Type Conversion1 : DataTypeConversion  OutDataTypeStr=single  SaturateOnIntegerOverflow=off  RndMeth=Floor
  Data Type Conversion2 : DataTypeConversion  OutDataTypeStr=single  SaturateOnIntegerOverflow=off  RndMeth=Floor
  MATLAB Function : MATLAB Function  TreatAsAtomicUnit=on
  SlalomMountPoseSet1 : sim3dlib/Simulation 3D Message Set  Priority=-1  SigName=WhiteSlalom5MountPoseSet  Ts=dt_sample  aMode=0
      settings: LibrarySourceBlock=aerolibsim3d/Simulation 3D Message Set
  SlalomPoseSet1 : sim3dlib/Simulation 3D Message Set  Priority=-1  SigName=WhiteSlalom5PoseSet  Ts=dt_sample  aMode=0
      settings: LibrarySourceBlock=aerolibsim3d/Simulation 3D Message Set
  World to UCS1 : Gain  Gain=transpose(M_WorldToUCS)  Multiplication=Matrix(u*K)
  drift : MATLAB Function  TreatAsAtomicUnit=on
  wires:
  WhiteSlalomPose/1 -> World to UCS1/1
  MATLAB Function/1(mountPose) -> Data Type Conversion2/1
  Data Type Conversion2/1 -> SlalomMountPoseSet1/1
  Data Type Conversion1/1 -> SlalomPoseSet1/1
  World to UCS1/1 -> drift/2(pose), MATLAB Function/1(mountedPose)
  In1/1 -> drift/1(t)
  drift/1(driftPose) -> Data Type Conversion1/1

== system VisionProcessingDesign_UCS/Set UCS Object Locations/Set Slalom Poses/Set White Slalom Pose 6 ==
  WhiteSlalomPose : Inport
  In1 : Inport  Port=2
  Data Type Conversion1 : DataTypeConversion  OutDataTypeStr=single  SaturateOnIntegerOverflow=off  RndMeth=Floor
  Data Type Conversion2 : DataTypeConversion  OutDataTypeStr=single  SaturateOnIntegerOverflow=off  RndMeth=Floor
  MATLAB Function : MATLAB Function  TreatAsAtomicUnit=on
  SlalomMountPoseSet1 : sim3dlib/Simulation 3D Message Set  Priority=-1  SigName=WhiteSlalom6MountPoseSet  Ts=dt_sample  aMode=0
      settings: LibrarySourceBlock=aerolibsim3d/Simulation 3D Message Set
  SlalomPoseSet1 : sim3dlib/Simulation 3D Message Set  Priority=-1  SigName=WhiteSlalom6PoseSet  Ts=dt_sample  aMode=0
      settings: LibrarySourceBlock=aerolibsim3d/Simulation 3D Message Set
  World to UCS1 : Gain  Gain=transpose(M_WorldToUCS)  Multiplication=Matrix(u*K)
  drift : MATLAB Function  TreatAsAtomicUnit=on
  wires:
  WhiteSlalomPose/1 -> World to UCS1/1
  MATLAB Function/1(mountPose) -> Data Type Conversion2/1
  Data Type Conversion2/1 -> SlalomMountPoseSet1/1
  Data Type Conversion1/1 -> SlalomPoseSet1/1
  World to UCS1/1 -> drift/2(pose), MATLAB Function/1(mountedPose)
  In1/1 -> drift/1(t)
  drift/1(driftPose) -> Data Type Conversion1/1

== matlab function VisionProcessingDesign_UCS/Set UCS Object Locations/Set Slalom Poses/Set Red Slalom Pose 2/MATLAB Function ==
  data: mountedPose input; mountPose output; ground_Z parameter
function mountPose = getMountPose(mountedPose,ground_Z)

mountPose = [mountedPose(1) mountedPose(2) (10 - ground_Z) 0 0 mountedPose(6)];

== matlab function VisionProcessingDesign_UCS/Set UCS Object Locations/Set Slalom Poses/Set Red Slalom Pose 3/MATLAB Function ==
  data: mountedPose input; mountPose output; ground_Z parameter
function mountPose = getMountPose(mountedPose,ground_Z)

mountPose = [mountedPose(1) mountedPose(2) (10 - ground_Z) 0 0 mountedPose(6)];

== matlab function VisionProcessingDesign_UCS/Set UCS Object Locations/Set Gate1 Pose/drift ==
  data: t input; pose input; driftPose output
function driftPose = drift(t,pose)
driftPose = toDriftedCoordinates(pose,t);

== matlab function VisionProcessingDesign_UCS/Set UCS Object Locations/Set Slalom Poses/Set Red Slalom Pose 1/drift ==
  data: t input; pose input; driftPose output
function driftPose = drift(t,pose)
driftPose = toDriftedCoordinates(pose,t);

== matlab function VisionProcessingDesign_UCS/Set UCS Object Locations/Set Slalom Poses/Set Red Slalom Pose 2/drift ==
  data: t input; pose input; driftPose output
function driftPose = drift(t,pose)
driftPose = toDriftedCoordinates(pose,t);

== matlab function VisionProcessingDesign_UCS/Set UCS Object Locations/Set Slalom Poses/Set Red Slalom Pose 3/drift ==
  data: t input; pose input; driftPose output
function driftPose = drift(t,pose)
driftPose = toDriftedCoordinates(pose,t);

== matlab function VisionProcessingDesign_UCS/Set UCS Object Locations/Set Slalom Poses/Set White Slalom Pose 1/drift ==
  data: t input; pose input; driftPose output
function driftPose = drift(t,pose)
driftPose = toDriftedCoordinates(pose,t);

== matlab function VisionProcessingDesign_UCS/Set UCS Object Locations/Set Slalom Poses/Set White Slalom Pose 2/drift ==
  data: t input; pose input; driftPose output
function driftPose = drift(t,pose)
driftPose = toDriftedCoordinates(pose,t);

== matlab function VisionProcessingDesign_UCS/Set UCS Object Locations/Set Slalom Poses/Set White Slalom Pose 3/drift ==
  data: t input; pose input; driftPose output
function driftPose = drift(t,pose)
driftPose = toDriftedCoordinates(pose,t);

== matlab function VisionProcessingDesign_UCS/Set UCS Object Locations/Set Slalom Poses/Set White Slalom Pose 4/drift ==
  data: t input; pose input; driftPose output
function driftPose = drift(t,pose)
driftPose = toDriftedCoordinates(pose,t);

== matlab function VisionProcessingDesign_UCS/Set UCS Object Locations/Set Slalom Poses/Set White Slalom Pose 5/drift ==
  data: t input; pose input; driftPose output
function driftPose = drift(t,pose)
driftPose = toDriftedCoordinates(pose,t);

== matlab function VisionProcessingDesign_UCS/Set UCS Object Locations/Set Slalom Poses/Set White Slalom Pose 6/drift ==
  data: t input; pose input; driftPose output
function driftPose = drift(t,pose)
driftPose = toDriftedCoordinates(pose,t);

== matlab function VisionProcessingDesign_UCS/MATLAB Function ==
  data: inputImage input; outputImage output
function outputImage = imageTransform(inputImage)
    for y = 1:1080
        for x = 1:1920
            r = double(inputImage(y,x,1));
            g = double(inputImage(y,x,2));
            b = double(inputImage(y,x,3));
            rg = g * 255 / r;
            rb = b * 255 / r;
            if 1 < (rb/250)^2 + (rg/200)^2
                inputImage(y,x,1) = 0;
                inputImage(y,x,2) = 0;
                inputImage(y,x,3) = 0;
            end
        end
    end
outputImage = inputImage;

== matlab function VisionProcessingDesign_UCS/Rectify Stereo Images ==
  settings: updateMethod=DISCRETE  sampleTime=1
  data: IL input; JL output size=[834 1491 3]; IR input; JR output size=[834 1491 3]; reprojectionMatrix output; stereo_params parameter Bus: stereo_bus
function [JL,JR,reprojectionMatrix] = rectify(IL, IR, stereo_params)

%intrinsics1 = cameraIntrinsics([1.067227033830202e+03, 1.068011951672645e+03], [9.600390418155606e+02,5.411961437864845e+02], [1080,1920], "RadialDistortion", [0.326188154119635,0.160769731106023]);
%intrinsics2 = cameraIntrinsics([1.067227033830202e+03, 1.068011951672645e+03], [9.600390418155606e+02,5.411961437864845e+02], [1080,1920], "RadialDistortion", [0.326188154119635,0.160769731106023]);
%poseCamera2 = rigidtform3d([0.999999486992860,6.654072773569351e-05,-0.001010735547931;-6.670699244698788e-05,0.999999984250571,-1.644659064942571e-04;0.001010724588331,1.645332452506317e-04,0.999999475682171],[-24.864043704444899,0.011387801702954,-0.025381336189953]);
%stereoParams = stereoParameters(intrinsics1, intrinsics2, poseCamera2);

s = stereo_params;
s.CameraParameters1.WorldUnits = 'centimeters';
s.CameraParameters2.WorldUnits = 'centimeters';

s.Version.Name = 'Computer Vision Toolbox';
s.Version.Version = '25.2';
s.Version.Release = '(R2025b)';
s.Version.Date = '28-Jul-2025';

s.RectificationParams.OutputView = 'valid';

stereoParams = stereoParameters(s);

JL = zeros(834,1491,3, "uint8");
JR = zeros(834,1491,3, "uint8");
[JL,JR,reprojectionMatrix] = rectifyStereoImages(IL,IR,stereoParams, "cubic");

== matlab function VisionProcessingDesign_UCS/MATLAB Function1 ==
  data: inputImage input; outputImage output
function outputImage = imageTransform(inputImage)
    for y = 1:1080
        for x = 1:1920
            r = double(inputImage(y,x,1));
            g = double(inputImage(y,x,2));
            b = double(inputImage(y,x,3));
            rg = g * 255 / r;
            rb = b * 255 / r;
            if 1 < (rb/250)^2 + (rg/200)^2
                inputImage(y,x,1) = 0;
                inputImage(y,x,2) = 0;
                inputImage(y,x,3) = 0;
            end
        end
    end
outputImage = inputImage;

== matlab function VisionProcessingDesign_UCS/MATLAB Function2 ==
  data: image input; newImage output uint8 size=[834 1491 3]
function newImage = edgeDetect(image)

grayImage = im2gray(image);
%blueImage = image(:,:,1);
newImage = uint8(zeros(834, 1491, 3));
[BW,threshOut] = edge(grayImage, 'canny', [0.07 0.12]);
graySobelImage = uint8(BW);
disp(threshOut)

newImage(:,:,1) = graySobelImage(:,:) * 255;
newImage(:,:,2) = graySobelImage(:,:) * 255;
newImage(:,:,3) = graySobelImage(:,:) * 255;
%{
corners = detectHarrisFeatures(grayImage).Location;
squareSize = 5;
dimensions = size(corners);
for i = 1:dimensions(1)
    x = round(corners(i, 1));
    y = round(corners(i, 2));
    if x <= 1920 - squareSize && x > squareSize && y <= 1080 - squareSize && y > squareSize
        for xi = (x - squareSize):(x + squareSize)
            for yi = (y - squareSize):(y + squareSize)
                grayImage(yi,xi) = 255;
            end
        end
    end
end
%}



%newImage = grayImage;

== matlab function VisionProcessingDesign_UCS/Dispairty Map ==
  data: grayImage1 input; grayImage2 input; disparityMap output size=[834 1491]
function disparityMap = fcn(grayImage1,grayImage2)

g1 = imgaussfilt(grayImage1,1);
g2 = imgaussfilt(grayImage2,1);
disparityRange = [5 93];
disparityMapIntermediate = disparitySGM(g1, g2, "DisparityRange", disparityRange, "UniquenessThreshold", 45);
disparityMap = uint8(disparityMapIntermediate);

== matlab function VisionProcessingDesign_UCS/MATLAB Function3 ==
  data: IL input; g1 output; IR input; g2 output; gray1 output uint8 size=[834 1491 3]; gray2 output uint8 size=[834 1491 3]
function [g1,g2, gray1, gray2] = grayImage(IL, IR)

g1 = uint8(rgb2gray(IL));
g2 = uint8(rgb2gray(IR));
[i,j] = size(g1);
gray1 = zeros(i,j,3,"uint8");
gray2 = zeros(i,j,3,"uint8");
gray1(:,:,1) = g1(:,:);
gray1(:,:,2) = g1(:,:);
gray1(:,:,3) = g1(:,:);
gray2(:,:,1) = g2(:,:);
gray2(:,:,2) = g2(:,:);
gray2(:,:,3) = g2(:,:);
g1 = IL(:,:,1);
g2 = IR(:,:,1);

== matlab function VisionProcessingDesign_UCS/MATLAB Function5 ==
  data: image input; newImage output uint8 size=[834 1491 3]
function newImage = edgeDetect(image)

grayImage = im2gray(image);
%blueImage = image(:,:,1);
newImage = uint8(zeros(834, 1491, 3));
graySobelImage = uint8(edge(grayImage, 'sobel'));

newImage(:,:,1) = graySobelImage(:,:) * 255;
newImage(:,:,2) = graySobelImage(:,:) * 255;
newImage(:,:,3) = graySobelImage(:,:) * 255;
%{
corners = detectHarrisFeatures(grayImage).Location;
squareSize = 5;
dimensions = size(corners);
for i = 1:dimensions(1)
    x = round(corners(i, 1));
    y = round(corners(i, 2));
    if x <= 1920 - squareSize && x > squareSize && y <= 1080 - squareSize && y > squareSize
        for xi = (x - squareSize):(x + squareSize)
            for yi = (y - squareSize):(y + squareSize)
                grayImage(yi,xi) = 255;
            end
        end
    end
end
%}



%newImage = grayImage;

== matlab function VisionProcessingDesign_UCS/Set UCS Object Locations/Set Slalom Poses/Set White Slalom Pose 1/MATLAB Function ==
  data: mountedPose input; mountPose output; ground_Z parameter
function mountPose = getMountPose(mountedPose,ground_Z)

mountPose = [mountedPose(1) mountedPose(2) (10 - ground_Z) 0 0 mountedPose(6)];

== matlab function VisionProcessingDesign_UCS/Set UCS Object Locations/Set Gate1 Pose/MATLAB Function ==
  data: mountedPose input; mountPose output; ground_Z parameter
function mountPose = getMountPose(mountedPose,ground_Z)

mountPose = [mountedPose(1) mountedPose(2) (10 - ground_Z) 0 0 mountedPose(6)];

== matlab function VisionProcessingDesign_UCS/Set UCS Object Locations/Set Gate1 Pose/MATLAB Function1 ==
  data: leftMountPose input; mountPose output
function mountPose = getMountPose(leftMountPose)

phi = leftMountPose(6) * pi / 180 + pi / 2;
xAdjust = 307 * cos(phi);
yAdjust = 307 * sin(phi);

mountPose = [(leftMountPose(1) + xAdjust) (leftMountPose(2) + yAdjust) leftMountPose(3) 0 0 leftMountPose(6)];

== matlab function VisionProcessingDesign_UCS/Set UCS Object Locations/Set Slalom Poses/Set White Slalom Pose 2/MATLAB Function ==
  data: mountedPose input; mountPose output; ground_Z parameter
function mountPose = getMountPose(mountedPose,ground_Z)

mountPose = [mountedPose(1) mountedPose(2) (10 - ground_Z) 0 0 mountedPose(6)];

== matlab function VisionProcessingDesign_UCS/Set UCS Object Locations/Set Slalom Poses/Set White Slalom Pose 3/MATLAB Function ==
  data: mountedPose input; mountPose output; ground_Z parameter
function mountPose = getMountPose(mountedPose,ground_Z)

mountPose = [mountedPose(1) mountedPose(2) (10 - ground_Z) 0 0 mountedPose(6)];

== matlab function VisionProcessingDesign_UCS/Set UCS Object Locations/Set Slalom Poses/Set White Slalom Pose 4/MATLAB Function ==
  data: mountedPose input; mountPose output; ground_Z parameter
function mountPose = getMountPose(mountedPose,ground_Z)

mountPose = [mountedPose(1) mountedPose(2) (10 - ground_Z) 0 0 mountedPose(6)];

== matlab function VisionProcessingDesign_UCS/Set UCS Object Locations/Set Slalom Poses/Set White Slalom Pose 5/MATLAB Function ==
  data: mountedPose input; mountPose output; ground_Z parameter
function mountPose = getMountPose(mountedPose,ground_Z)

mountPose = [mountedPose(1) mountedPose(2) (10 - ground_Z) 0 0 mountedPose(6)];

== matlab function VisionProcessingDesign_UCS/Set UCS Object Locations/Set Slalom Poses/Set White Slalom Pose 6/MATLAB Function ==
  data: mountedPose input; mountPose output; ground_Z parameter
function mountPose = getMountPose(mountedPose,ground_Z)

mountPose = [mountedPose(1) mountedPose(2) (10 - ground_Z) 0 0 mountedPose(6)];

== matlab function VisionProcessingDesign_UCS/Set UCS Object Locations/Set Slalom Poses/Set Red Slalom Pose 1/MATLAB Function ==
  data: mountedPose input; mountPose output; ground_Z parameter
function mountPose = getMountPose(mountedPose,ground_Z)

mountPose = [mountedPose(1) mountedPose(2) (10 - ground_Z) 0 0 mountedPose(6)];
